simulink model "PIL_motore"  (R2023b)
settings: Solver=FixedStepDiscrete  StartTime=0.0  StopTime=50  FixedStep=Ts  RelTol=1e-3  EnableMultiTasking=on
values from neighbouring files (symbols this model uses):
  kr = -1/(C*inv(A-B*K_tilde(1:3))*B)    [controller_tuning.m]    (also in progetto.m = -1/(C*inv(A-B*K)*B); tuning.m)
  sys_discrete = c2d(sys_continuos,0.005,'tustin')    [observer.m]
  Ts = 0.005    [attempt.m]    (also in model_approximation.m; tuning.m)
undefined symbols (not defined in the file or in its folder): K_tilde
libraries: mbedblockslib x3, cstblocks x2, stm_qeplib x1, eeStairGenerator x1
settings Model: ExtModeTrigDuration=10  Creator=giova  LastModifiedBy=giova
settings OptimizationCC: EnhancedBackFolding=on  PassReuseOutputArgsAs=Individual arguments  ZeroExternalMemoryAtStartup=off  ZeroInternalMemoryAtStartup=off  MaxStackSize=64  OptimizeBlockOrder=speed  DifferentSizesBufferReuse=on  OptimizationCustomize=off  EfficientTunableParamExpr=on
settings DebuggingCC: ParameterTunabilityLossMsg=error
settings HardwareCC: ProdBitPerPointer=32  ProdBitPerSizeT=32  ProdBitPerPtrDiffT=32  ProdLargestAtomicInteger=Long  ProdLargestAtomicFloat=Double  ProdWordSize=32  ProdLongLongMode=on  ProdHWDeviceType=ARM Compatible->ARM Cortex
settings SFSimCC: MATLABDynamicMemAlloc=off
settings RTWCC: Description=Embedded Coder  SystemTargetFile=ert.tlc  HardwareBoard=STM32 Nucleo F401RE  TemplateMakefile=ert_default_tmf  Toolchain=GNU Tools for ARM Embedded Processors
settings CodeAppCC: ForceParamTrailComments=on  IgnoreCustomStorageClasses=off  OperatorAnnotations=on  SimulinkDataObjDesc=on  SFDataObjDesc=on  InsertBlockDesc=on
settings ERTTargetCC: ExtModeTransport=3  ExtModeStaticAlloc=on  ExtModeStaticAllocSize=2000  ExtModeMexFile=ext_xcp  ExtModeIntrfLevel=Level2 - Open

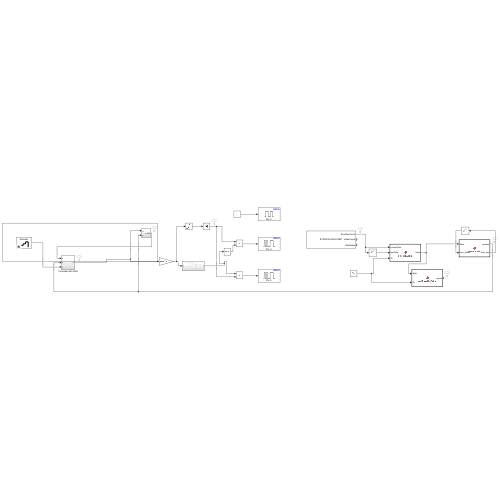
[thumbnail: Simulink's stored preview of the top-level diagram]
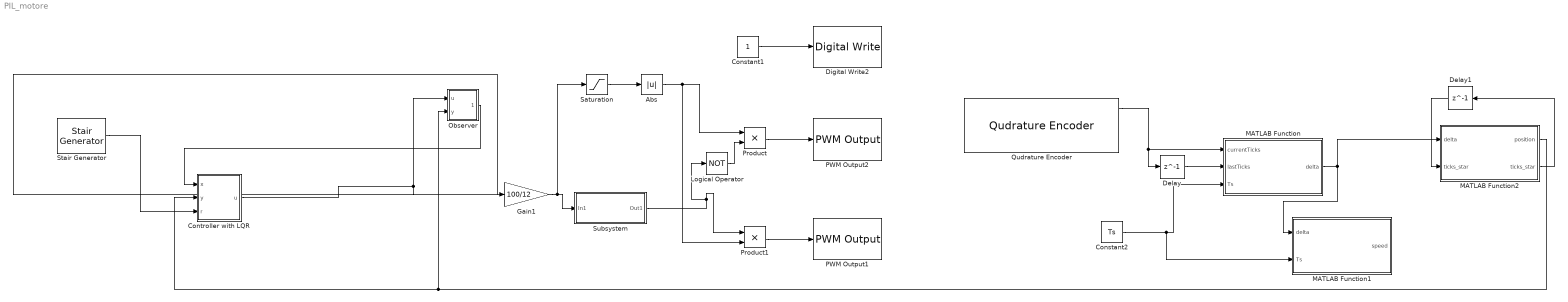
== system PIL_motore ==
  Abs : Abs  SaturateOnIntegerOverflow=off
  Constant1 : Constant
  Constant2 : Constant  Value=Ts
  Controller with LQR : Subsystem
  Delay : Delay  DelayLength=1  SampleTime=Ts
  Delay1 : Delay  DelayLength=1  SampleTime=Ts
  Digital Write2 : mbedblockslib/Digital Write  Pin=2  Direction=output
      settings: LibrarySourceBlock=stmnucleorootlib/Common/Digital Write
  Gain1 : Gain  Gain=100/12
  Logical Operator : Logic  Operator=NOT  AllPortsSameDT=off  OutDataTypeStr=boolean
  MATLAB Function : MATLAB Function  TreatAsAtomicUnit=on
  MATLAB Function1 : MATLAB Function  TreatAsAtomicUnit=on
  MATLAB Function2 : MATLAB Function  TreatAsAtomicUnit=on
  Observer : Subsystem
  PWM Output1 : mbedblockslib/PWM Output  Pin=5  EnableInputFrequency=off  InitialFrequency=2000  InitialDutyCycle=50  NotificationType=None
      settings: LibrarySourceBlock=stmnucleorootlib/Common/PWM Output
  PWM Output2 : mbedblockslib/PWM Output  Pin=4  EnableInputFrequency=off  InitialFrequency=2000  InitialDutyCycle=50  NotificationType=None
      settings: LibrarySourceBlock=stmnucleorootlib/Common/PWM Output
  Product : Product
  Product1 : Product
  Qudrature Encoder : stm_qeplib/Qudrature Encoder  SampleTime=Ts
  Saturation : Saturate  UpperLimit=100  LowerLimit=-100
  Stair Generator : eeStairGenerator/Stair Generator  LabelModeActiveChoice=Discrete  TimeInput=[0 10 20 30]  AmplitudeInput=[2 4 2*pi 0]  SampleTime=Ts  RepeatPattern=off  OutDataTypeStr=double
      settings: LibrarySourceBlock=ee_sl_lib/General Control/Stair Generator
  Subsystem : Subsystem
  wires:
  Observer/1(x_hat) -> Controller with LQR/1(x)
  Controller with LQR/1(u) -> Observer/1(u), Gain1/1
  Subsystem/1(Out1) -> Logical Operator/1, Product1/1
  Delay/1 -> MATLAB Function/2(lastTicks)
  Constant2/1 -> MATLAB Function1/2(Ts), MATLAB Function/3(Ts)
  Constant1/1 -> Digital Write2/1
  Product1/1 -> PWM Output1/1
  Qudrature Encoder/1 -> MATLAB Function/1(currentTicks), Delay/1
  Product/1 -> PWM Output2/1
  Abs/1 -> Product1/2, Product/1
  MATLAB Function/1(delta) -> MATLAB Function1/1(delta), MATLAB Function2/1(delta)
  Gain1/1 -> Saturation/1, Subsystem/1(In1)
  Logical Operator/1 -> Product/2
  Saturation/1 -> Abs/1
  Delay1/1 -> MATLAB Function2/2("ticks_star ")
  MATLAB Function2/2(ticks_star) -> Delay1/1
  MATLAB Function2/1(position) -> Observer/2(y), Controller with LQR/2(y)
  Stair Generator/1 -> Controller with LQR/3(r)

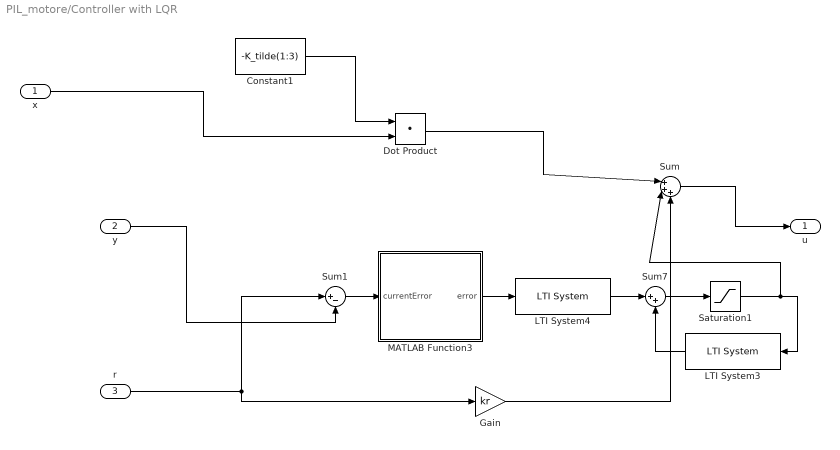
== system PIL_motore/Controller with LQR ==
  x : Inport
  y : Inport  Port=2
  r : Inport  Port=3
  Constant1 : Constant  Value=-K_tilde(1:3)
  Dot Product : DotProduct  OutDataTypeStr=Inherit: Inherit via internal rule
  Gain : Gain  Gain=kr
  LTI System3 : cstblocks/LTI System  sys=z_antiwindupFunc  IC=[]  PadeOrder=0
  LTI System4 : cstblocks/LTI System  sys=z_Q_Gamma  IC=[]  PadeOrder=0
  MATLAB Function3 : MATLAB Function  TreatAsAtomicUnit=on
  Saturation1 : Saturate  UpperLimit=12  LowerLimit=-12
  Sum : Sum  Inputs=|+++
  Sum1 : Sum  Inputs=|+-
  Sum7 : Sum  Inputs=|++
  u : Outport
  wires:
  r/1 -> Sum1/1, Gain/1
  Gain/1 -> Sum/3
  Constant1/1 -> Dot Product/1
  Sum/1 -> u/1
  x/1 -> Dot Product/2
  y/1 -> Sum1/2
  Dot Product/1 -> Sum/1
  Sum1/1 -> MATLAB Function3/1(currentError)
  Sum7/1 -> Saturation1/1
  LTI System3/1 -> Sum7/2
  Saturation1/1 -> Sum/2, LTI System3/1
  LTI System4/1 -> Sum7/1
  MATLAB Function3/1(error) -> LTI System4/1

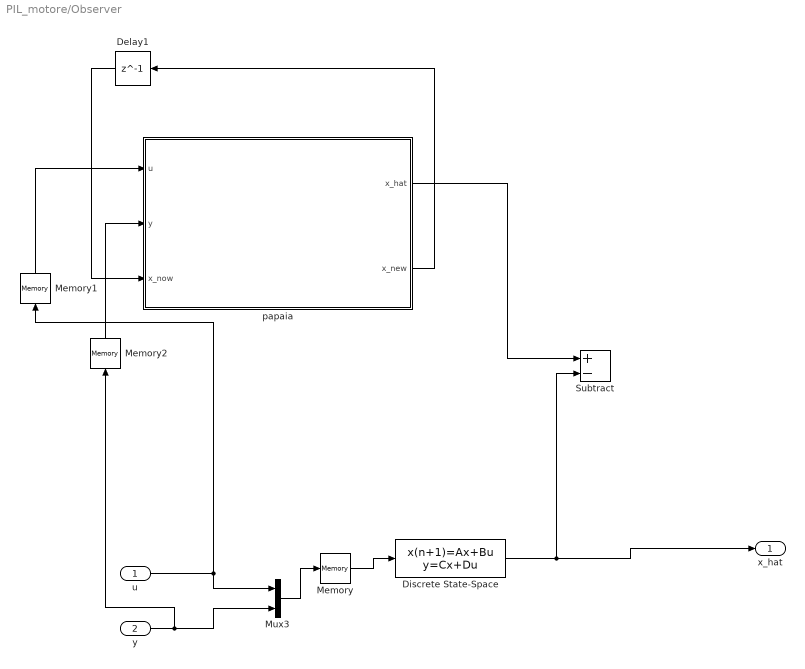
== system PIL_motore/Observer ==
  u : Inport
  y : Inport  Port=2
  Delay1 : Delay  DelayLength=1  InitialCondition=[0.0 ;0.0 ;0.0]  SampleTime=Ts
  Discrete State-Space : DiscreteStateSpace  A=sys_discrete.A  B=sys_discrete.B  C=sys_discrete.C  D=sys_discrete.D  SampleTime=Ts
  Memory : Memory
  Memory1 : Memory
  Memory2 : Memory
  Mux3 : Mux  Inputs=2
  Subtract : Sum  Inputs=+-
  papaia : MATLAB Function  TreatAsAtomicUnit=on
  x_hat : Outport
  wires:
  y/1 -> Mux3/2, Memory2/1
  u/1 -> Mux3/1, Memory1/1
  Mux3/1 -> Memory/1
  Memory/1 -> Discrete State-Space/1
  Discrete State-Space/1 -> x_hat/1, Subtract/2
  Memory2/1 -> papaia/2(y)
  Memory1/1 -> papaia/1(u)
  papaia/2(x_new) -> Delay1/1
  Delay1/1 -> papaia/3(x_now)
  papaia/1(x_hat) -> Subtract/1

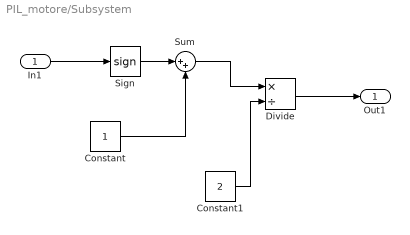
== system PIL_motore/Subsystem ==
  In1 : Inport
  Constant : Constant
  Constant1 : Constant  Value=2
  Divide : Product  Inputs=*/
  Sign : Signum
  Sum : Sum  Inputs=|++
  Out1 : Outport
  wires:
  Constant/1 -> Sum/2
  In1/1 -> Sign/1
  Sign/1 -> Sum/1
  Sum/1 -> Divide/1
  Constant1/1 -> Divide/2
  Divide/1 -> Out1/1

== matlab function PIL_motore/MATLAB Function1 ==
  data: delta input; speed output; Ts input
function speed = getSpeedByDelta(delta, Ts)
    speed = delta*60/(8400*Ts)

end

== matlab function PIL_motore/MATLAB Function ==
  data: currentTicks input; delta output; lastTicks input; Ts input
function delta = getTicksDelta(currentTicks, lastTicks, Ts)

currentTicks = double(currentTicks);
lastTicks = double(lastTicks);

if abs(currentTicks-lastTicks) <= ceil(12600*Ts)
    delta = currentTicks-lastTicks
else
    if lastTicks > currentTicks
        delta = currentTicks+2^16-1-lastTicks;
    else
        delta = currentTicks-2^16+1-lastTicks;
    end
end

end

== matlab function PIL_motore/MATLAB Function2 ==
  data: delta input; position output; ticks_star input; ticks_star output
function [position,ticks_star] = getPosition(delta, ticks_star)
    
    ticks_star = double(ticks_star+delta);

    position = 2*pi*ticks_star/(8400);

    
end

== matlab function PIL_motore/Controller with LQR/MATLAB Function3 ==
  data: currentError input; error output
function error = getErrorPos(currentError)

error=currentError;
if (currentError>pi)
    error = currentError-2*pi;
end

if(currentError<-pi)
    error = currentError + 2*pi;
end

end

== matlab function PIL_motore/Observer/papaia ==
  data: u input; x_hat output; y input; x_new output; x_now input
function [x_hat,x_new]= fcn(u, y, x_now)
A = [0.9323301716064688  -11.678660637721487    0.039014496138124237;
    0.0027413091396064947    0.1183557159613379    5.5348095481874759e-5;
   -0.0068954979109303533   -2.8131155992845822    0.8383381318909956];

B = [-0.0040505355062536866    2.0794225090756346;
   -5.7463109393787418e-6    0.15697955665449895;
    0.036784001382597235    0.50088414067706177];
    
C = [0.96616508580323435  -5.8393303188607444    0.019507248069062118;
    0.0013706545698032474    0.559177857980669    2.767404774093738e-5;
   -0.0034477489554651771  -1.4065577996422911    0.91916906594549774];

D = [-0.0020252677531268433    1.0397112545378173;
   -2.8731554696893709e-6   0.078489778327249474;
    0.018392000691298618   0.25044207033853089];

x1 = x_now(1);
x2 = x_now(2);
x3 = x_now(3);

x1_stimato = C(1) * x1 + C(4) * x2 + C(7) * x3 + D(1) * u + D(4) * y;
x2_stimato = C(2) * x1 + C(5) * x2 + C(8) * x3 + D(2) * u + D(5) * y;
x3_stimato = C(3) * x1 + C(6) * x2 + C(9) * x3 + D(3) * u + D(6) * y;

x1_new = A(1) * x1 + A(4) * x2 + A(7) * x3 + B(1) * u + B(4) * y;
x2_new = A(2) * x1 + A(5) * x2 + A(8) * x3 + B(2) * u + B(5) * y;
x3_new = A(3) * x1 + A(6) * x2 + A(9) * x3 + B(3) * u + B(6) * y;


x_new = [x1_new ;x2_new ;x3_new];
x_hat = [x1_stimato ;x2_stimato ;x3_stimato];
